simulink model "Assignment_2_3K04_Updated_2"  (R2022b)
settings: Solver=FixedStepAuto  StartTime=0.0  StopTime=1  FixedStep=1e-3  RelTol=1e-3  EnableMultiTasking=on
undefined symbols (not defined in the file): A0, A1, D0, D1, D10, D11, D12, D13, D2, D3, D4, D5, D6, D7, D8, D9, PTA0, PTA1, PTA2, PTB2, PTB23, PTB3, PTB9, PTC16, PTC17, PTC2, PTC3, PTC4, PTD0, PTD1, PTD2, PTD3
libraries: frdmk64flib x22, dspstat3 x1
settings Model: ExtModeTrigDuration=5  Creator=Stephen Oh  LastModifiedBy=Mehak
settings SolverCC: AlgebraicLoopSolver=TrustRegion
settings OptimizationCC: EnhancedBackFolding=on  PassReuseOutputArgsAs=Individual arguments  ZeroExternalMemoryAtStartup=off  ZeroInternalMemoryAtStartup=off  MaxStackSize=64  OptimizeBlockOrder=speed  DifferentSizesBufferReuse=on  OptimizationCustomize=off  EfficientTunableParamExpr=on
settings DebuggingCC: ParameterPrecisionLossMsg=none  ParameterTunabilityLossMsg=error  UnconnectedInputMsg=warning  UnconnectedOutputMsg=warning  UnconnectedLineMsg=warning  SFMachineParentedDataDiag=warning
settings HardwareCC: ProdBitPerPointer=32  ProdBitPerSizeT=32  ProdBitPerPtrDiffT=32  ProdLargestAtomicInteger=Long  ProdLargestAtomicFloat=Double  ProdWordSize=32  ProdHWDeviceType=ARM Compatible->ARM Cortex
settings ModelReferenceCC: EnableRefExpFcnMdlSchedulingChecks=on
settings SFSimCC: MATLABDynamicMemAlloc=off
settings RTWCC: Description=Embedded Coder  SystemTargetFile=ert.tlc  HardwareBoard=NXP FRDM-K64F  TLCOptions="-aInlineSetEventsForThisBaseRateFcn=TLC_FALSE -aSuppressMultiTaskScheduler=TLC_FALSE  -aRateBasedStepFcn=0"  TemplateMakefile=ert_default_tmf  Toolchain=GNU Tools for ARM Embedded Processors
settings CodeAppCC: ForceParamTrailComments=on  IgnoreCustomStorageClasses=off  OperatorAnnotations=on  SimulinkDataObjDesc=on  SFDataObjDesc=on  InsertBlockDesc=on

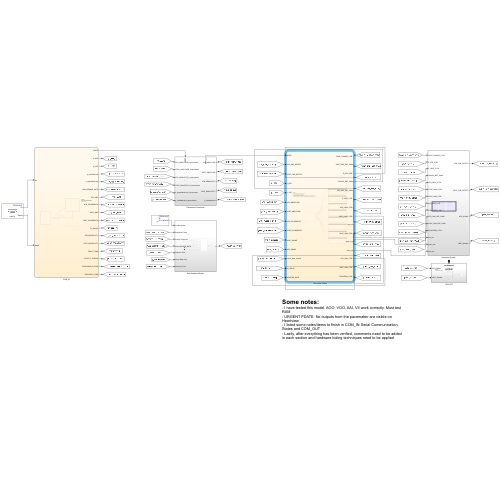
[thumbnail: Simulink's stored preview of the top-level diagram]
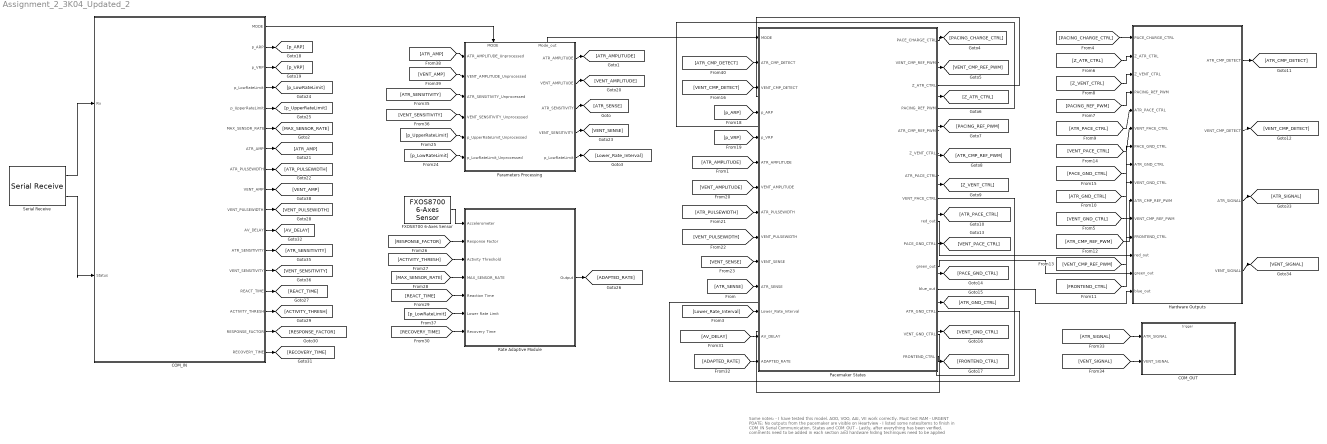
== system Assignment_2_3K04_Updated_2 ==
  note: Some notes:
      | - I have tested this model. AOO, VOO, AAI, VII work correctly. Must test RAM
      | - URGENT PDATE: No outputs from the pacemaker are visible on Heartview
      | - I listed some notes/items to finish in COM_IN Serial Communication, States and COM_OUT
      | - Lastly, after everything has been verified, comments need to be added in each section and hardware hiding techniques need to be applied
  COM_IN : Stateflow chart  TreatAsAtomicUnit=on
      settings: PortSchema="{\"entries\":[{\"content\":{\"sides\":[{\"content\":{\"connectorIds\":[\"In1\",\"In2\"]},\"type\":\"ConnectorPlacement.EquallySpacedRectSide\",\"uuid\":\"1aa50ecf-3a03-4bd0-8c8d-e8c42c1df160\"},{\"content\":{\"connectorIds\":[\"Out1\",\"Out2\",\"Out5\",\"Out3\",\"Out4\",\"Out10\",\"Out6\",\"Out9\",\"Out7\",\"Out8\",\"Out11\",\"Out17\",\"Out12\",\"Out13\",\"Out14\",\"Out15\",\"Out16\"],\"side\":\"RIGHT\"},\"type\":\"ConnectorPlacement.EquallySpacedRectSide\",\"uuid\":\"11f4d1ba-79ca-4268-a70d-42de969d73ee\"},{\"content\":{\"connectorIds\":[],\"side\":\"TOP\"},\"type\":\"ConnectorPlacement.EquallySpacedRectSide\",\"uuid\":\"6aafc352-a891-4eaa-b435-c000b57676be\"}]},\"type\":\"ConnectorPlacement.EquallySpacedConnector\",\"uuid\":\"60cf4415-29e1-4f60-bb1b-ba03cc79869a\"}],\"packageUris\":[\"http://schema.mathworks.com/mf0/Connector/R2020b\"],\"version\":\"1.0\"}"
  COM_OUT : Subsystem  TreatAsAtomicUnit=on
  FXOS8700 6-Axes Sensor : frdmk64flib/FXOS8700 6-Axes Sensor  Activesensor=Accelerometer only  ODR=800Hz  HybridODR=400Hz  Accelfullrange=-4g to +4g  SampleTime=-1
  Hardware Outputs : Subsystem
  Pacemaker States : Stateflow chart  TreatAsAtomicUnit=on
      settings: PortSchema="{\"entries\":[{\"content\":{\"sides\":[{\"content\":{\"connectorIds\":[\"In2\",\"In3\",\"In4\",\"In5\",\"In6\",\"In7\",\"In8\",\"In9\",\"In10\",\"In11\",\"In12\",\"In1\",\"In13\",\"In14\"]},\"type\":\"ConnectorPlacement.EquallySpacedRectSide\",\"uuid\":\"15e03f69-5c25-4f3e-b3fb-d71978e552f4\"},{\"content\":{\"connectorIds\":[\"Out7\",\"Out12\",\"Out4\",\"Out8\",\"Out10\",\"Out5\",\"Out9\",\"Out3\",\"Out15\",\"Out6\",\"Out14\",\"Out13\",\"Out1\",\"Out2\",\"Out11\"],\"side\":\"RIGHT\"},\"type\":\"ConnectorPlacement.EquallySpacedRectSide\",\"uuid\":\"02171bf1-edb1-4b01-9e56-a8642c556ed6\"},{\"content\":{\"connectorIds\":[],\"side\":\"TOP\"},\"type\":\"ConnectorPlacement.EquallySpacedRectSide\",\"uuid\":\"cc6b5506-3435-4740-9e3f-4dfe15d30bff\"}]},\"type\":\"ConnectorPlacement.EquallySpacedConnector\",\"uuid\":\"0ad55da7-1e65-48d0-a0a4-2620ffa94320\"}],\"packageUris\":[\"http://schema.mathworks.com/mf0/Connector/R2020b\"],\"version\":\"1.0\"}"
  Parameters Processing : Subsystem
      settings: PortSchema="{\"entries\":[{\"content\":{\"sides\":[{\"content\":{\"connectorIds\":[\"In1\",\"In2\",\"In3\",\"In4\",\"In5\",\"In6\"]},\"type\":\"ConnectorPlacement.EquallySpacedRectSide\",\"uuid\":\"651e63ca-28f2-42bd-8706-028901d11c05\"},{\"content\":{\"connectorIds\":[\"Out1\",\"Out2\",\"Out3\",\"Out4\",\"Out5\"],\"side\":\"RIGHT\"},\"type\":\"ConnectorPlacement.EquallySpacedRectSide\",\"uuid\":\"490f658c-59fe-438c-accc-92ccac1dea65\"},{\"content\":{\"connectorIds\":[\"In7\",\"Out6\"],\"side\":\"TOP\"},\"type\":\"ConnectorPlacement.EquallySpacedRectSide\",\"uuid\":\"f083c363-f6a9-47da-81a0-6b2bc7e9f843\"}]},\"type\":\"ConnectorPlacement.EquallySpacedConnector\",\"uuid\":\"6dd41c46-d50c-4376-aa14-7404fb0d5350\"}],\"packageUris\":[\"http://schema.mathworks.com/mf0/Connector/R2020b\"],\"version\":\"1.0\"}"
  Rate Adaptive Module : Subsystem
  Serial Receive : frdmk64flib/Serial Receive  SCIModule=0  Baudrate=uint32(9600)  Parity=None  StopBits=1  HardwareFlowControl=None  ByteOrder=LittleEndian  DataType=uint8  DataLength=66  BlockingMode=off  OutputStatus=on  SampleTime=-1
  wires:
  [Lower_Rate_Interval] -> Pacemaker States/1(Lower_Rate_Interval)
  [ATR_GND_CTRL] -> Hardware Outputs/8(ATR_GND_CTRL)
  [PACING_REF_PWM] -> Hardware Outputs/4(PACING_REF_PWM)
  [Z_VENT_CTRL] -> Hardware Outputs/3(Z_VENT_CTRL)
  [ATR_PACE_CTRL] -> Hardware Outputs/5(ATR_PACE_CTRL)
  Hardware Outputs/2(VENT_CMP_DETECT) -> [VENT_CMP_DETECT]
  [PACE_GND_CTRL] -> Hardware Outputs/7(PACE_GND_CTRL)
  [FRONTEND_CTRL] -> Hardware Outputs/12(FRONTEND_CTRL)
  [VENT_GND_CTRL] -> Hardware Outputs/9(VENT_GND_CTRL)
  [Z_ATR_CTRL] -> Hardware Outputs/2(Z_ATR_CTRL)
  [VENT_PACE_CTRL] -> Hardware Outputs/6(VENT_PACE_CTRL)
  [ATR_CMP_REF_PWM] -> Hardware Outputs/10(ATR_CMP_REF_PWM)
  [VENT_CMP_REF_PWM] -> Hardware Outputs/11(VENT_CMP_REF_PWM)
  [PACING_CHARGE_CTRL] -> Hardware Outputs/1(PACE_CHARGE_CTRL)
  Hardware Outputs/1(ATR_CMP_DETECT) -> [ATR_CMP_DETECT]
  [VENT_CMP_DETECT] -> Pacemaker States/4(VENT_CMP_DETECT)
  [p_ARP] -> Pacemaker States/5(p_ARP)
  [p_VRP] -> Pacemaker States/6(p_VRP)
  [ATR_CMP_DETECT] -> Pacemaker States/3(ATR_CMP_DETECT)
  [ATR_AMPLITUDE] -> Pacemaker States/7(ATR_AMPLITUDE)
  [VENT_AMPLITUDE] -> Pacemaker States/8(VENT_AMPLITUDE)
  [ATR_PULSEWIDTH] -> Pacemaker States/9(ATR_PULSEWIDTH)
  [VENT_PULSEWIDTH] -> Pacemaker States/10(VENT_PULSEWIDTH)
  Parameters Processing/1(ATR_AMPLITUDE) -> [ATR_AMPLITUDE]
  Parameters Processing/5(p_LowRateLimit) -> [Lower_Rate_Interval]
  Pacemaker States/3(VENT_PACE_CTRL) -> [VENT_PACE_CTRL]
  Pacemaker States/9(ATR_PACE_CTRL) -> [ATR_PACE_CTRL]
  Pacemaker States/7(PACE_CHARGE_CTRL) -> [PACING_CHARGE_CTRL]
  Pacemaker States/12(VENT_CMP_REF_PWM) -> [VENT_CMP_REF_PWM]
  Pacemaker States/4(Z_ATR_CTRL) -> [Z_ATR_CTRL]
  Pacemaker States/8(PACING_REF_PWM) -> [PACING_REF_PWM]
  Pacemaker States/10(ATR_CMP_REF_PWM) -> [ATR_CMP_REF_PWM]
  Pacemaker States/5(Z_VENT_CTRL) -> [Z_VENT_CTRL]
  Pacemaker States/6(PACE_GND_CTRL) -> [PACE_GND_CTRL]
  Pacemaker States/1(ATR_GND_CTRL) -> [ATR_GND_CTRL]
  Pacemaker States/2(VENT_GND_CTRL) -> [VENT_GND_CTRL]
  Pacemaker States/11(FRONTEND_CTRL) -> [FRONTEND_CTRL]
  [ATR_SENSE] -> Pacemaker States/12(ATR_SENSE)
  [VENT_SENSE] -> Pacemaker States/11(VENT_SENSE)
  Serial Receive/1 -> COM_IN/1(Rx)
  Serial Receive/2 -> COM_IN/2(Status)
  COM_IN/1(MODE) -> Parameters Processing/7(MODE)
  Parameters Processing/6(Mode_out) -> Pacemaker States/2(MODE)
  Parameters Processing/2(VENT_AMPLITUDE) -> [VENT_AMPLITUDE]
  [p_UpperRateLimit] -> Parameters Processing/5(p_UpperRateLimit_Unprocessed)
  COM_IN/11(AV_DELAY) -> [AV_DELAY]
  [AV_DELAY] -> Pacemaker States/13(AV_DELAY)
  [ADAPTED_RATE] -> Pacemaker States/14(ADAPTED_RATE)
  Parameters Processing/3(ATR_SENSITIVITY) -> [ATR_SENSE]
  Parameters Processing/4(VENT_SENSITIVITY) -> [VENT_SENSE]
  FXOS8700 6-Axes Sensor/1 -> Rate Adaptive Module/1(Accelerometer)
  Rate Adaptive Module/1(Output) -> [ADAPTED_RATE]
  [RESPONSE_FACTOR] -> Rate Adaptive Module/2(Response Factor)
  [ACTIVITY_THRESH] -> Rate Adaptive Module/3(Activity Threshold)
  [MAX_SENSOR_RATE] -> Rate Adaptive Module/4(MAX_SENSOR_RATE)
  [REACT_TIME] -> Rate Adaptive Module/5(Reaction Time)
  [p_LowRateLimit] -> Parameters Processing/6(p_LowRateLimit_Unprocessed)
  [RECOVERY_TIME] -> Rate Adaptive Module/7(Recovery Time)
  Hardware Outputs/3(ATR_SIGNAL) -> [ATR_SIGNAL]
  Hardware Outputs/4(VENT_SIGNAL) -> [VENT_SIGNAL]
  [ATR_SIGNAL] -> COM_OUT/1(ATR_SIGNAL)
  [VENT_SIGNAL] -> COM_OUT/2(VENT_SIGNAL)
  [ATR_SENSITIVITY] -> Parameters Processing/3(ATR_SENSITIVITY_Unprocessed)
  [VENT_SENSITIVITY] -> Parameters Processing/4(VENT_SENSITIVITY_Unprocessed)
  [p_LowRateLimit] -> Rate Adaptive Module/6(Lower Rate Limit)
  COM_IN/3(p_LowRateLimit) -> [p_LowRateLimit]
  COM_IN/4(p_UpperRateLimit) -> [p_UpperRateLimit]
  COM_IN/5(p_VRP) -> [p_VRP]
  COM_IN/2(p_ARP) -> [p_ARP]
  COM_IN/10(MAX_SENSOR_RATE) -> [MAX_SENSOR_RATE]
  COM_IN/17(ATR_SENSITIVITY) -> [ATR_SENSITIVITY]
  COM_IN/12(VENT_SENSITIVITY) -> [VENT_SENSITIVITY]
  COM_IN/9(ATR_PULSEWIDTH) -> [ATR_PULSEWIDTH]
  COM_IN/8(VENT_PULSEWIDTH) -> [VENT_PULSEWIDTH]
  COM_IN/6(ATR_AMP) -> [ATR_AMP]
  COM_IN/7(VENT_AMP) -> [VENT_AMP]
  COM_IN/13(REACT_TIME) -> [REACT_TIME]
  COM_IN/14(ACTIVITY_THRESH) -> [ACTIVITY_THRESH]
  COM_IN/15(RESPONSE_FACTOR) -> [RESPONSE_FACTOR]
  COM_IN/16(RECOVERY_TIME) -> [RECOVERY_TIME]
  [ATR_AMP] -> Parameters Processing/1(ATR_AMPLITUDE_Unprocessed)
  [VENT_AMP] -> Parameters Processing/2(VENT_AMPLITUDE_Unprocessed)
  Pacemaker States/15(red_out) -> Hardware Outputs/13(red_out)
  Pacemaker States/13(blue_out) -> Hardware Outputs/15(blue_out)
  Pacemaker States/14(green_out) -> Hardware Outputs/14(green_out)

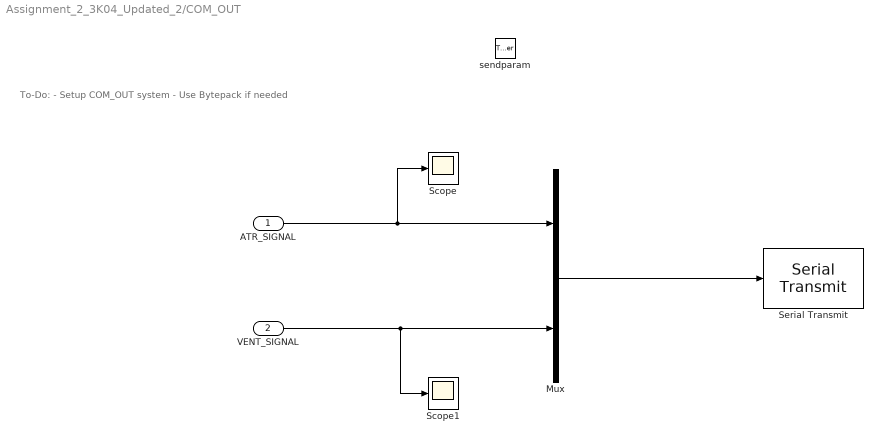
== system Assignment_2_3K04_Updated_2/COM_OUT ==
  note: To-Do:
      | - Setup COM_OUT system
      | - Use Bytepack if needed
  ATR_SIGNAL : Inport  OutDataTypeStr=double
  VENT_SIGNAL : Inport  Port=2  OutDataTypeStr=double
  sendparam : TriggerPort  TriggerType=function-call  IsSimulinkFunction=on  FunctionName=sendparam  VariantControl=(inherit)  PortDimensions=1
  Mux : Mux  Inputs=2
  Scope : Scope
  Scope1 : Scope
  Serial Transmit : frdmk64flib/Serial Transmit  SCIModule=0  Baudrate=uint32(9600)  Parity=None  StopBits=1  HardwareFlowControl=None  ByteOrder=LittleEndian  BlockingMode=on  OutputStatus=off
  wires:
  ATR_SIGNAL/1 -> Scope/1, Mux/1
  VENT_SIGNAL/1 -> Scope1/1, Mux/2
  Mux/1 -> Serial Transmit/1

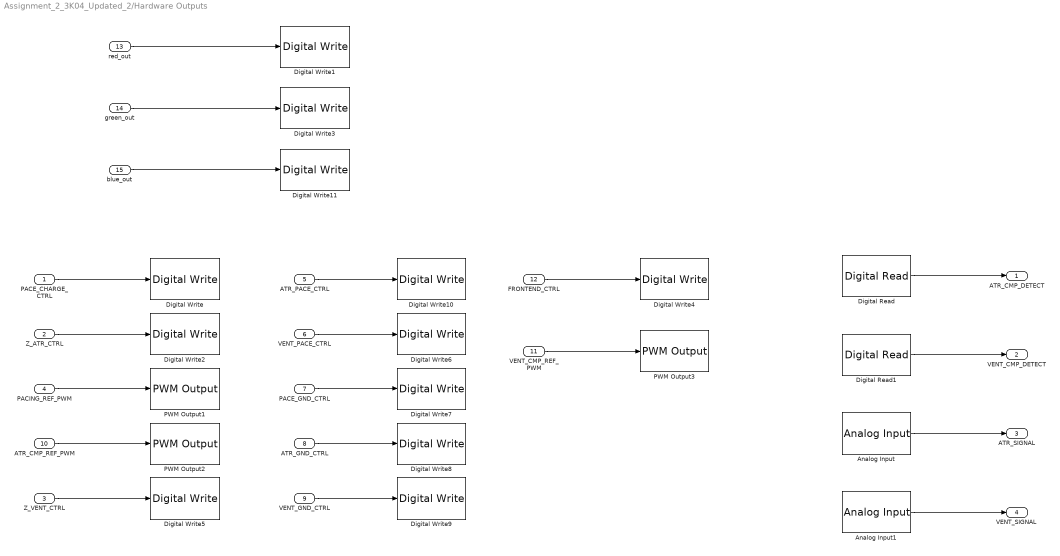
== system Assignment_2_3K04_Updated_2/Hardware Outputs ==
  PACE_CHARGE_CTRL : Inport
  Z_ATR_CTRL : Inport  Port=2
  Z_VENT_CTRL : Inport  Port=3
  PACING_REF_PWM : Inport  Port=4
  ATR_PACE_CTRL : Inport  Port=5
  VENT_PACE_CTRL : Inport  Port=6
  PACE_GND_CTRL : Inport  Port=7
  ATR_GND_CTRL : Inport  Port=8
  VENT_GND_CTRL : Inport  Port=9
  ATR_CMP_REF_PWM : Inport  Port=10
  VENT_CMP_REF_PWM : Inport  Port=11
  FRONTEND_CTRL : Inport  Port=12
  red_out : Inport  Port=13
  green_out : Inport  Port=14
  blue_out : Inport  Port=15
  Analog Input : frdmk64flib/Analog Input  Whichpin=PTB2 (A0)  SampleTime=-1
  Analog Input1 : frdmk64flib/Analog Input  Whichpin=PTB3 (A1)  SampleTime=-1
  Digital Read : frdmk64flib/Digital Read  Whichpin=PTC16 (D0)  SampleTime=-1
  Digital Read1 : frdmk64flib/Digital Read  Whichpin=PTC17 (D1)  SampleTime=-1
  Digital Write : frdmk64flib/Digital Write  Whichpin=PTB9 (D2)
  Digital Write1 : frdmk64flib/Digital Write  Whichpin=RED_LED
  Digital Write10 : frdmk64flib/Digital Write  Whichpin=PTA0 (D8)
  Digital Write11 : frdmk64flib/Digital Write  Whichpin=BLUE_LED
  Digital Write2 : frdmk64flib/Digital Write  Whichpin=PTB23 (D4)
  Digital Write3 : frdmk64flib/Digital Write  Whichpin=GREEN_LED
  Digital Write4 : frdmk64flib/Digital Write  Whichpin=PTD1 (D13)
  Digital Write5 : frdmk64flib/Digital Write  Whichpin=PTC3 (D7)
  Digital Write6 : frdmk64flib/Digital Write  Whichpin=PTC4 (D9)
  Digital Write7 : frdmk64flib/Digital Write  Whichpin=PTD0 (D10)
  Digital Write8 : frdmk64flib/Digital Write  Whichpin=PTD2 (D11)
  Digital Write9 : frdmk64flib/Digital Write  Whichpin=PTD3 (D12)
  PWM Output1 : frdmk64flib/PWM Output  Whichpin=PTA2 (D5)  InitialFrequency=2000  InitialDutyCycle=0
  PWM Output2 : frdmk64flib/PWM Output  Whichpin=PTC2 (D6)  InitialFrequency=2000  InitialDutyCycle=0
  PWM Output3 : frdmk64flib/PWM Output  Whichpin=PTA1 (D3)  InitialFrequency=2000  InitialDutyCycle=0
  ATR_CMP_DETECT : Outport
  VENT_CMP_DETECT : Outport  Port=2
  ATR_SIGNAL : Outport  Port=3  OutDataTypeStr=double
  VENT_SIGNAL : Outport  Port=4  OutDataTypeStr=double
  wires:
  Analog Input1/1 -> VENT_SIGNAL/1
  Analog Input/1 -> ATR_SIGNAL/1
  FRONTEND_CTRL/1 -> Digital Write4/1
  Digital Read1/1 -> VENT_CMP_DETECT/1
  PACE_GND_CTRL/1 -> Digital Write7/1
  VENT_CMP_REF_PWM/1 -> PWM Output3/1
  Z_VENT_CTRL/1 -> Digital Write5/1
  PACE_CHARGE_CTRL/1 -> Digital Write/1
  PACING_REF_PWM/1 -> PWM Output1/1
  ATR_GND_CTRL/1 -> Digital Write8/1
  VENT_PACE_CTRL/1 -> Digital Write6/1
  ATR_CMP_REF_PWM/1 -> PWM Output2/1
  VENT_GND_CTRL/1 -> Digital Write9/1
  Digital Read/1 -> ATR_CMP_DETECT/1
  Z_ATR_CTRL/1 -> Digital Write2/1
  ATR_PACE_CTRL/1 -> Digital Write10/1
  blue_out/1 -> Digital Write11/1
  red_out/1 -> Digital Write1/1
  green_out/1 -> Digital Write3/1

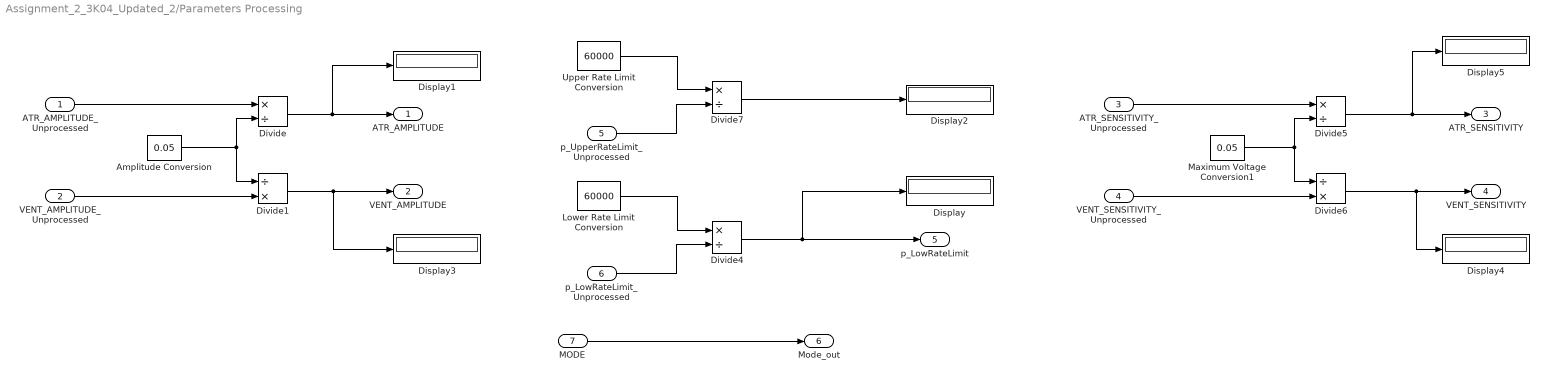
== system Assignment_2_3K04_Updated_2/Parameters Processing ==
  ATR_AMPLITUDE_Unprocessed : Inport  OutDataTypeStr=single
  VENT_AMPLITUDE_Unprocessed : Inport  Port=2  OutDataTypeStr=single
  ATR_SENSITIVITY_Unprocessed : Inport  Port=3  OutDataTypeStr=single
  VENT_SENSITIVITY_Unprocessed : Inport  Port=4  OutDataTypeStr=single
  p_UpperRateLimit_Unprocessed : Inport  Port=5  OutDataTypeStr=single
  p_LowRateLimit_Unprocessed : Inport  Port=6  OutDataTypeStr=single
  MODE : Inport  Port=7
  Amplitude Conversion : Constant  Value=0.05  OutDataTypeStr=single
  Display{,1..5} (6 alike) : Display
  Divide : Product  Inputs=*/  OutDataTypeStr=single
  Divide1 : Product  Inputs=/*  OutDataTypeStr=single
  Divide4 : Product  Inputs=*/  OutDataTypeStr=single  RndMeth=Nearest
  Divide5 : Product  Inputs=*/  OutDataTypeStr=single
  Divide6 : Product  Inputs=/*  OutDataTypeStr=single
  Divide7 : Product  Inputs=*/  OutDataTypeStr=single  RndMeth=Nearest
  Lower Rate Limit Conversion : Constant  Value=60000  OutDataTypeStr=single
  Maximum Voltage Conversion1 : Constant  Value=0.05  OutDataTypeStr=single
  Upper Rate Limit Conversion : Constant  Value=60000  OutDataTypeStr=single
  ATR_AMPLITUDE : Outport  OutDataTypeStr=single
  VENT_AMPLITUDE : Outport  Port=2  OutDataTypeStr=single
  ATR_SENSITIVITY : Outport  Port=3  OutDataTypeStr=single
  VENT_SENSITIVITY : Outport  Port=4  OutDataTypeStr=single
  p_LowRateLimit : Outport  Port=5  OutDataTypeStr=single
  Mode_out : Outport  Port=6
  wires:
  Divide5/1 -> Display5/1, ATR_SENSITIVITY/1
  Divide7/1 -> Display2/1
  Upper Rate Limit Conversion/1 -> Divide7/1
  p_UpperRateLimit_Unprocessed/1 -> Divide7/2
  Lower Rate Limit Conversion/1 -> Divide4/1
  Divide1/1 -> Display3/1, VENT_AMPLITUDE/1
  ATR_SENSITIVITY_Unprocessed/1 -> Divide5/1
  p_LowRateLimit_Unprocessed/1 -> Divide4/2
  Maximum Voltage Conversion1/1 -> Divide6/1, Divide5/2
  Divide/1 -> Display1/1, ATR_AMPLITUDE/1
  Divide4/1 -> p_LowRateLimit/1, Display/1
  VENT_AMPLITUDE_Unprocessed/1 -> Divide1/2
  VENT_SENSITIVITY_Unprocessed/1 -> Divide6/2
  ATR_AMPLITUDE_Unprocessed/1 -> Divide/1
  Divide6/1 -> Display4/1, VENT_SENSITIVITY/1
  Amplitude Conversion/1 -> Divide1/1, Divide/2
  MODE/1 -> Mode_out/1

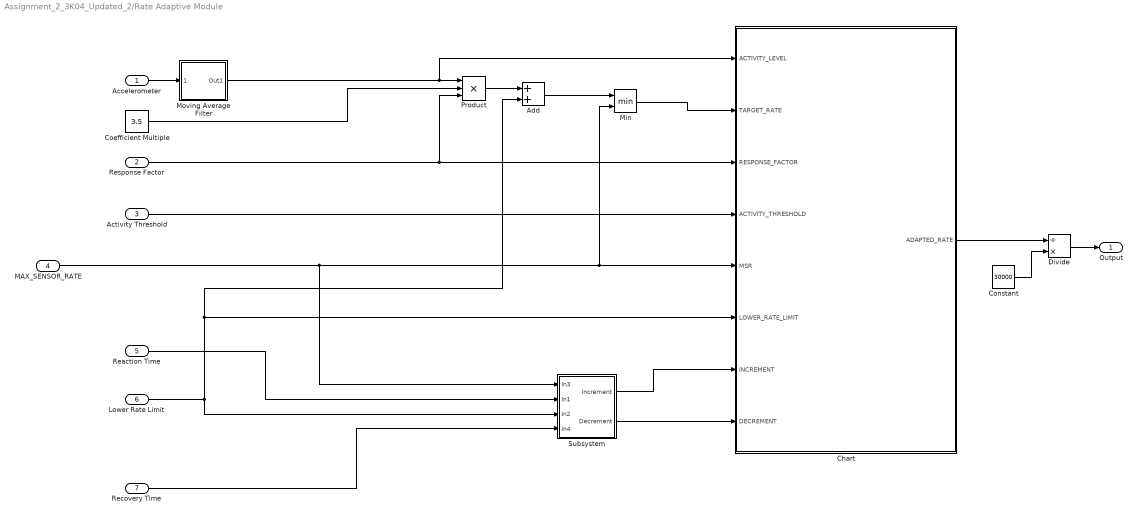
== system Assignment_2_3K04_Updated_2/Rate Adaptive Module ==
  Accelerometer : Inport
  Response Factor : Inport  Port=2
  Activity Threshold : Inport  Port=3
  MAX_SENSOR_RATE : Inport  Port=4
  Reaction Time : Inport  Port=5
  Lower Rate Limit : Inport  Port=6
  Recovery Time : Inport  Port=7
  Add : Sum
  Chart : Stateflow chart  TreatAsAtomicUnit=on
      settings: PortSchema="{\"entries\":[{\"content\":{\"sides\":[{\"content\":{\"connectorIds\":[\"In1\",\"In3\",\"In2\",\"In6\",\"In8\",\"In7\",\"In4\",\"In5\"]},\"type\":\"ConnectorPlacement.EquallySpacedRectSide\",\"uuid\":\"efebee7e-2c09-4b25-ba04-904f72c011ed\"},{\"content\":{\"connectorIds\":[\"Out1\"],\"side\":\"RIGHT\"},\"type\":\"ConnectorPlacement.EquallySpacedRectSide\",\"uuid\":\"6322cc63-1b7a-423a-b49b-7b27e71e0c32\"},{\"content\":{\"connectorIds\":[],\"side\":\"TOP\"},\"type\":\"ConnectorPlacement.EquallySpacedRectSide\",\"uuid\":\"daf2dbd4-7676-46e9-bb01-958bd0e2e14e\"}]},\"type\":\"ConnectorPlacement.EquallySpacedConnector\",\"uuid\":\"43c3c7b3-b94c-45f5-b310-1a430cfb2b71\"}],\"packageUris\":[\"http://schema.mathworks.com/mf0/Connector/19700101\"],\"version\":\"1.0\"}"
  Coefficient Multiple : Constant  Value=3.5
  Constant : Constant  Value=30000
  Divide : Product  Inputs=/*
  Min : MinMax  Inputs=2
  Moving Average Filter : Subsystem
  Product : Product  Inputs=3
  Subsystem : Subsystem
  Output : Outport
  wires:
  Recovery Time/1 -> Subsystem/4(In4)
  MAX_SENSOR_RATE/1 -> Subsystem/1(In3), Min/2, Chart/8(MSR)
  Subsystem/1(Increment) -> Chart/4(INCREMENT)
  Activity Threshold/1 -> Chart/6(ACTIVITY_THRESHOLD)
  Response Factor/1 -> Product/3, Chart/2(RESPONSE_FACTOR)
  Lower Rate Limit/1 -> Subsystem/3(In2), Chart/7(LOWER_RATE_LIMIT), Add/2
  Add/1 -> Min/1
  Product/1 -> Add/1
  Min/1 -> Chart/3(TARGET_RATE)
  Reaction Time/1 -> Subsystem/2(In1)
  Subsystem/2(Decrement) -> Chart/5(DECREMENT)
  Chart/1(ADAPTED_RATE) -> Divide/1
  Coefficient Multiple/1 -> Product/2
  Divide/1 -> Output/1
  Constant/1 -> Divide/2
  Moving Average Filter/1(Out1) -> Chart/1(ACTIVITY_LEVEL), Product/1
  Accelerometer/1 -> Moving Average Filter/1(Accelerometer)

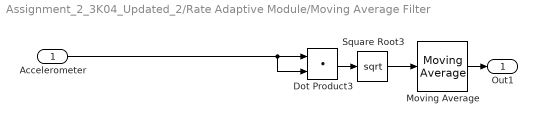
== system Assignment_2_3K04_Updated_2/Rate Adaptive Module/Moving Average Filter ==
  Accelerometer : Inport
  Dot Product3 : DotProduct  OutDataTypeStr=Inherit: Inherit via internal rule
  Moving Average : dspstat3/Moving Average  Method=Sliding window  ForgettingFactorPort=off  SpecifyWindowLength=on  WindowLength=500  OverlapLength=499  AllowArbitraryInputLength=off  ForgettingFactor=0.9  SimulateUsing=Code generation
  Square Root3 : Sqrt
  Out1 : Outport
  wires:
  Accelerometer/1 -> Dot Product3/2, Dot Product3/1
  Dot Product3/1 -> Square Root3/1
  Square Root3/1 -> Moving Average/1
  Moving Average/1 -> Out1/1

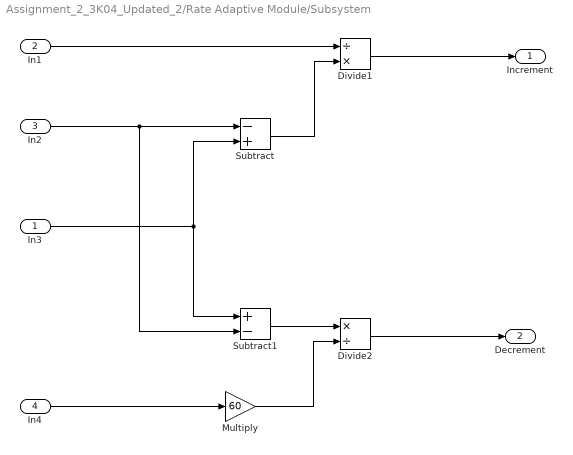
== system Assignment_2_3K04_Updated_2/Rate Adaptive Module/Subsystem ==
  In3 : Inport  OutDataTypeStr=single
  In1 : Inport  Port=2  OutDataTypeStr=single
  In2 : Inport  Port=3  OutDataTypeStr=single
  In4 : Inport  Port=4  OutDataTypeStr=single
  Divide1 : Product  Inputs=/*  RndMeth=Ceiling
  Divide2 : Product  Inputs=*/  RndMeth=Ceiling  SaturateOnIntegerOverflow=on
  Multiply : Gain  Gain=60
  Subtract : Sum  Inputs=-+
  Subtract1 : Sum  Inputs=+-
  Increment : Outport  OutDataTypeStr=single
  Decrement : Outport  Port=2  OutDataTypeStr=single
  wires:
  Multiply/1 -> Divide2/2
  In2/1 -> Subtract1/2, Subtract/1
  In3/1 -> Subtract/2, Subtract1/1
  Divide1/1 -> Increment/1
  In1/1 -> Divide1/1
  Subtract1/1 -> Divide2/1
  Subtract/1 -> Divide1/2
  In4/1 -> Multiply/1
  Divide2/1 -> Decrement/1

== stateflow chart Assignment_2_3K04_Updated_2/COM_IN ==
  state SET_PARAM
    % Uses serial input to assign values to the parameters
    entry:
    MODE = Rx(1);
    p_ARP = typecast(Rx(2:5), "single");
    p_VRP = typecast(Rx(6:9), "single");
    p_LowRateLimit = typecast(Rx(10:13), "single");
    p_UpperRateLimit = typecast(Rx(14:17), "single");
    MAX_SENSOR_RATE = typecast(Rx(18:21), "single");
    ATR_AMP = typecast(Rx(22:25), "single");
    ATR_PULSEWIDTH = typecast(Rx(26:29), "single");
    VENT_AMP = typecast(Rx(30:33), "single");
    VENT_PULSEWIDTH = typecast(Rx(34:37), "single");
    AV_DELAY = typecast(Rx(38:41), "single");
    ATR_SENSITIVITY = typecast(Rx(42:45), "single");
    VENT_SENSITIVITY = typecast(Rx(46:49), "single");
    REACT_TIME = typecast(Rx(50:53), "single");
    ACTIVITY_THRESH = typecast(Rx(54:57), "single");
    RESPONSE_FACTOR = typecast(Rx(58:61), "single");
    RECOVERY_TIME = typecast(Rx(62:65), "single");
  note: To-Do:
      | - Set number of transmitted bytes
      | - Update SET_PARAM with values
      | - Verify Fuction
  state INITIAL
    % Set the initial values of parameters
    entry:
    MODE = 5;
    p_ARP = 250;
    p_VRP = 320;
    p_LowRateLimit = 60;
    p_UpperRateLimit = 120;
    MAX_SENSOR_RATE = 120;
    ATR_AMP = 3.5;
    ATR_PULSEWIDTH = 1;
    VENT_AMP = 3.5;
    VENT_PULSEWIDTH = 1;
    AV_DELAY = 150;
    ATR_SENSITIVITY = 4;
    VENT_SENSITIVITY = 4;
    REACT_TIME = 30;
    ACTIVITY_THRESH = 1.1;
    RESPONSE_FACTOR = 8;
    RECOVERY_TIME = 5;
  state STANDBY
    % Wait for COM
  state ECHO_PARAM [commented out]
    entry:
    % Sends back the current value of the parameters
    sendparam();
  SET_PARAM -> STANDBY
  (default) -> INITIAL
  (junction 13) -> SET_PARAM : [Rx(66) == hex2dec('00')]
  (junction 12) -> STANDBY [order 2]
  INITIAL -> STANDBY
  STANDBY -> (junction 12) : [Status == 0]
  (junction 12) -> (junction 13) [order 1]
  (junction 13) -> ECHO_PARAM [commented out] : [Rx(2) == hex2dec('22')]
  ECHO_PARAM -> STANDBY [commented out]
  data: Rx input uint8; Status input uint8; MODE output uint8; p_ARP output single; p_LowRateLimit output single; p_UpperRateLimit output single; p_VRP output single; ATR_AMP output single; VENT_AMP output single; VENT_PULSEWIDTH output single; ATR_PULSEWIDTH output single; MAX_SENSOR_RATE output single; AV_DELAY output single; VENT_SENSITIVITY output single; REACT_TIME output single; ACTIVITY_THRESH output single; RESPONSE_FACTOR output single; RECOVERY_TIME output single; ATR_SENSITIVITY output single

== stateflow chart Assignment_2_3K04_Updated_2/Rate Adaptive Module/Chart ==
  state RateSelect
    entry:
    ADAPTED_RATE = LOWER_RATE_LIMIT
  state Increment
    entry:
    ADAPTED_RATE = ADAPTED_RATE + INCREMENT
  state TargetRateAchieved
  state Decrement
    entry:
    ADAPTED_RATE = ADAPTED_RATE - DECREMENT
  Increment -> Increment [order 2] : after(1000, msec) [ACTIVITY_LEVEL > ACTIVITY_THRESHOLD]
  (default) -> RateSelect
  Increment -> TargetRateAchieved [order 1] : [ADAPTED_RATE >= TARGET_RATE ]
  RateSelect -> Increment [order 1] : [ACTIVITY_LEVEL > ACTIVITY_THRESHOLD]
  RateSelect -> RateSelect [order 2] : [ACTIVITY_LEVEL < ACTIVITY_THRESHOLD]
  Decrement -> RateSelect [order 3] : [ADAPTED_RATE <= LOWER_RATE_LIMIT]
  Decrement -> Increment [order 1] : after(1000, msec) [ACTIVITY_LEVEL > ACTIVITY_THRESHOLD]
  Increment -> Decrement [order 3] : after(1000, msec) [ACTIVITY_LEVEL < ACTIVITY_THRESHOLD]
  TargetRateAchieved -> Decrement : [ACTIVITY_LEVEL < ACTIVITY_THRESHOLD]
  Decrement -> Decrement [order 2] : after(1000, msec) [ACTIVITY_LEVEL < ACTIVITY_THRESHOLD]
  data: ACTIVITY_LEVEL input; RESPONSE_FACTOR input; ADAPTED_RATE output; TARGET_RATE input; INCREMENT input; DECREMENT input; ACTIVITY_THRESHOLD input; LOWER_RATE_LIMIT input; MSR input

== stateflow chart Assignment_2_3K04_Updated_2/Pacemaker States ==
  state AOO
    state Charging
      entry:
      %
      % Charging capacitor C22
      ATR_PACE_CTRL = LOW
      VENT_PACE_CTRL = LOW
      PACING_REF_PWM = ATR_AMPLITUDE
      PACE_CHARGE_CTRL = HIGH
      %
      % Release of capacitor C21 into ground
      PACE_GND_CTRL = HIGH
      VENT_PACE_CTRL = LOW
      Z_ATR_CTRL = LOW
      Z_VENT_CTRL = LOW
      ATR_PACE_CTRL = LOW
      ATR_GND_CTRL = HIGH
      VENT_GND_CTRL = LOW
      red_out = 1;
      green_out = 0;
      blue_out = 0;
    state Discharging
      entry:
      %
      % Charge release of capacitor C22 into C21
      PACE_CHARGE_CTRL = LOW
      PACE_GND_CTRL = HIGH
      VENT_PACE_CTRL = LOW
      VENT_GND_CTRL = LOW
      Z_VENT_CTRL = LOW
      Z_ATR_CTRL = LOW
      ATR_GND_CTRL = LOW
      ATR_PACE_CTRL = HIGH
    (default) -> AOO.Charging
    AOO.Charging -> AOO.Discharging : after(delayINTERVAL, msec)
    AOO.Discharging -> AOO.Charging : after(delayATR_PULSEWIDTH, msec)
  note: To-Do:
      | - AOO, VOO, AAI, VVI work as intended
      | - Uncertain about AOOR and VOOR
      | - AAIR and VVIR work as intended (double-check on another pacemaker)
      | - Finally, add comments + organize
      | - If there is enough time remaining, implement DDDR (else delete AV_DELAY)
  state VOO
    state Charging
      entry:
      %
      % Charging capacitor C22
      ATR_PACE_CTRL = LOW
      VENT_PACE_CTRL = LOW
      PACING_REF_PWM = VENT_AMPLITUDE
      PACE_CHARGE_CTRL = HIGH
      %
      % Charge release of capacitor C21 into ground
      PACE_GND_CTRL = HIGH
      VENT_PACE_CTRL = LOW
      Z_ATR_CTRL = LOW
      Z_VENT_CTRL = LOW
      ATR_PACE_CTRL = LOW
      ATR_GND_CTRL = LOW
      VENT_GND_CTRL = HIGH
      red_out = 0;
      green_out = 0;
      blue_out = 1;
    state Discharging
      entry:
      %
      % Charge release of capacitor C22 into C21
      PACE_CHARGE_CTRL = LOW
      PACE_GND_CTRL = HIGH
      ATR_PACE_CTRL = LOW
      ATR_GND_CTRL = LOW
      Z_VENT_CTRL = LOW
      Z_ATR_CTRL = LOW
      VENT_GND_CTRL = LOW
      VENT_PACE_CTRL = HIGH
    (default) -> VOO.Charging
    VOO.Charging -> VOO.Discharging : after(delayINTERVAL, msec)
    VOO.Discharging -> VOO.Charging : after(delayVENT_PULSEWIDTH, msec)
  state AAI
    state Transition
      % Check for intrinsic pulse
    state Discharging
      entry:
      %
      % Charge release of capacitor C22 into C21
      PACE_CHARGE_CTRL = LOW
      PACE_GND_CTRL = HIGH
      VENT_PACE_CTRL = LOW
      VENT_GND_CTRL = LOW
      Z_VENT_CTRL = LOW
      Z_ATR_CTRL = LOW
      ATR_GND_CTRL = LOW
      ATR_PACE_CTRL = HIGH
    state Charging
      entry:
      %
      % Turn sensing on
      FRONTEND_CTRL = HIGH
      ATR_CMP_REF_PWM = ATR_SENSE
      %
      % Charging capacitor C22
      ATR_PACE_CTRL = LOW
      VENT_PACE_CTRL = LOW
      PACING_REF_PWM = ATR_AMPLITUDE
      PACE_CHARGE_CTRL = HIGH
      %
      % Charge release of capacitor C21 into ground
      PACE_GND_CTRL = HIGH
      VENT_PACE_CTRL = LOW
      Z_ATR_CTRL = LOW
      Z_VENT_CTRL = LOW
      ATR_PACE_CTRL = LOW
      ATR_GND_CTRL = HIGH
      VENT_GND_CTRL = LOW
    AAI.Transition -> AAI.Discharging [order 1] : after(delayINTERVAL-delayARP, msec)
    AAI.Transition -> AAI.Charging [order 2] : [ATR_CMP_DETECT == HIGH]
    AAI.Charging -> AAI.Transition : after(delayARP, msec)
    (default) -> AAI.Charging
    AAI.Discharging -> AAI.Charging : after(delayATR_PULSEWIDTH, msec)
  state VVI
    state Transition
      % Check for intrinsic pulse
    state Charging
      entry:
      %
      % Turn sensing on
      FRONTEND_CTRL = HIGH
      VENT_CMP_REF_PWM = VENT_SENSE
      %
      % Charging capacitor C22
      ATR_PACE_CTRL = LOW
      VENT_PACE_CTRL = LOW
      PACING_REF_PWM = VENT_AMPLITUDE
      PACE_CHARGE_CTRL = HIGH
      %
      % Charge release of capacitor C21 into ground
      PACE_GND_CTRL = HIGH
      VENT_PACE_CTRL = LOW
      Z_ATR_CTRL = LOW
      Z_VENT_CTRL = LOW
      ATR_PACE_CTRL = LOW
      ATR_GND_CTRL = LOW
      VENT_GND_CTRL = HIGH
    state Discharging
      entry:
      %
      % Charge release of capacitor C22 into C21
      PACE_CHARGE_CTRL = LOW
      PACE_GND_CTRL = HIGH
      ATR_PACE_CTRL = LOW
      ATR_GND_CTRL = LOW
      Z_VENT_CTRL = LOW
      Z_ATR_CTRL = LOW
      VENT_GND_CTRL = LOW
      VENT_PACE_CTRL = HIGH
    VVI.Transition -> VVI.Discharging [order 1] : after(delayINTERVAL-delayVRP, msec)
    VVI.Transition -> VVI.Charging [order 2] : [VENT_CMP_DETECT == HIGH]
    VVI.Charging -> VVI.Transition : after(delayVRP, msec)
    (default) -> VVI.Charging
    VVI.Discharging -> VVI.Charging : after(delayVENT_PULSEWIDTH, msec)
  state ModeSelect
  state AOOR
    state Charging
      entry:
      %
      % Charging capacitor C22
      ATR_PACE_CTRL = LOW
      VENT_PACE_CTRL = LOW
      PACING_REF_PWM = ATR_AMPLITUDE
      PACE_CHARGE_CTRL = HIGH
      %
      % Charge release of capacitor C21 into ground
      PACE_GND_CTRL = HIGH
      VENT_PACE_CTRL = LOW
      Z_ATR_CTRL = LOW
      Z_VENT_CTRL = LOW
      ATR_PACE_CTRL = LOW
      ATR_GND_CTRL = HIGH
      VENT_GND_CTRL = LOW
    state Discharging
      entry:
      %
      %Charge release of capacitor C22 into C21
      PACE_CHARGE_CTRL = LOW
      PACE_GND_CTRL = HIGH
      VENT_PACE_CTRL = LOW
      VENT_GND_CTRL = LOW
      Z_VENT_CTRL = LOW
      Z_ATR_CTRL = LOW
      ATR_GND_CTRL = LOW
      ATR_PACE_CTRL = HIGH
    (default) -> AOOR.Charging
    AOOR.Charging -> AOOR.Discharging : after(ADAPTED_RATE, msec)
    AOOR.Discharging -> AOOR.Charging : after(delayATR_PULSEWIDTH, msec)
  state VOOR
    state Discharging
      entry:
      %
      % Charge release of capacitor C22 into C21
      PACE_CHARGE_CTRL = LOW
      PACE_GND_CTRL = HIGH
      ATR_PACE_CTRL = LOW
      ATR_GND_CTRL = LOW
      Z_VENT_CTRL = LOW
      Z_ATR_CTRL = LOW
      VENT_GND_CTRL = LOW
      VENT_PACE_CTRL = HIGH
    state Charging
      entry:
      %
      % Charging capacitor C22
      ATR_PACE_CTRL = LOW
      VENT_PACE_CTRL = LOW
      PACING_REF_PWM = VENT_AMPLITUDE
      PACE_CHARGE_CTRL = HIGH
      %
      % Charge release of capacitor C21 into ground
      PACE_GND_CTRL = HIGH
      VENT_PACE_CTRL = LOW
      Z_ATR_CTRL = LOW
      Z_VENT_CTRL = LOW
      ATR_PACE_CTRL = LOW
      ATR_GND_CTRL = LOW
      VENT_GND_CTRL = HIGH
      red_out = 0;
      green_out = 1;
      blue_out = 0;
    (default) -> VOOR.Charging
    VOOR.Charging -> VOOR.Discharging : after(ADAPTED_RATE, msec)
    VOOR.Discharging -> VOOR.Charging : after(delayVENT_PULSEWIDTH, msec)
  state AAIR
    state Transition
      % Check for intrinsic pulse
    state Discharging
      entry:
      %
      % Charge release of capacitor C22 into C21
      PACE_CHARGE_CTRL = LOW
      PACE_GND_CTRL = HIGH
      VENT_PACE_CTRL = LOW
      VENT_GND_CTRL = LOW
      Z_VENT_CTRL = LOW
      Z_ATR_CTRL = LOW
      ATR_GND_CTRL = LOW
      ATR_PACE_CTRL = HIGH
    state Charging
      entry:
      %
      % Turn sensing on
      FRONTEND_CTRL = HIGH
      ATR_CMP_REF_PWM = ATR_SENSE
      %
      % Charging capacitor C22
      ATR_PACE_CTRL = LOW
      VENT_PACE_CTRL = LOW
      PACING_REF_PWM = ATR_AMPLITUDE
      PACE_CHARGE_CTRL = HIGH
      %
      % Charge release of capacitor C21 into ground
      PACE_GND_CTRL = HIGH
      VENT_PACE_CTRL = LOW
      Z_ATR_CTRL = LOW
      Z_VENT_CTRL = LOW
      ATR_PACE_CTRL = LOW
      ATR_GND_CTRL = HIGH
      VENT_GND_CTRL = LOW
    AAIR.Transition -> AAIR.Discharging [order 1] : after(ADAPTED_RATE - delayARP, msec)
    AAIR.Transition -> AAIR.Charging [order 2] : [ATR_CMP_DETECT == HIGH]
    AAIR.Charging -> AAIR.Transition : after(delayARP, msec)
    (default) -> AAIR.Charging
    AAIR.Discharging -> AAIR.Charging : after(delayATR_PULSEWIDTH, msec)
  state VVIR
    state Transition
      % Check for intrinsic pulse
    state Charging
      entry:
      %
      % Turn sensing on
      FRONTEND_CTRL = HIGH
      VENT_CMP_REF_PWM = VENT_SENSE
      %
      % Charging capacitor C22
      ATR_PACE_CTRL = LOW
      VENT_PACE_CTRL = LOW
      PACING_REF_PWM = VENT_AMPLITUDE
      PACE_CHARGE_CTRL = HIGH
      % Charge release of capacitor C21 into ground
      PACE_GND_CTRL = HIGH
      VENT_PACE_CTRL = LOW
      Z_ATR_CTRL = LOW
      Z_VENT_CTRL = LOW
      ATR_PACE_CTRL = LOW
      ATR_GND_CTRL = LOW
      VENT_GND_CTRL = HIGH
    state Discharging
      entry:
      %
      % Charge release of capacitor C22 into C21
      PACE_CHARGE_CTRL = LOW
      PACE_GND_CTRL = HIGH
      ATR_PACE_CTRL = LOW
      ATR_GND_CTRL = LOW
      Z_VENT_CTRL = LOW
      Z_ATR_CTRL = LOW
      VENT_GND_CTRL = LOW
      VENT_PACE_CTRL = HIGH
    VVIR.Transition -> VVIR.Discharging [order 1] : after(ADAPTED_RATE-delayVRP, msec)
    VVIR.Transition -> VVIR.Charging [order 2] : [VENT_CMP_DETECT == HIGH]
    VVIR.Charging -> VVIR.Transition : after(delayVRP, msec)
    (default) -> VVIR.Charging
    VVIR.Discharging -> VVIR.Charging : after(delayVENT_PULSEWIDTH, msec)
  ModeSelect -> AOO [order 1] : [MODE == 0]
  AOO -> ModeSelect : [MODE ~= 0]
  ModeSelect -> VOO [order 2] : [MODE == 1]
  VOO -> ModeSelect : [MODE ~= 1]
  ModeSelect -> AAI [order 3] : [MODE == 2]
  AAI -> ModeSelect : [MODE ~= 2]
  (default) -> ModeSelect : {delayINTERVAL = Lower_Rate_Interval/2,
      |  delayAV_DELAY = AV_DELAY/2,
      |  delayARP = p_ARP/2,
      |  delayVRP = p_VRP/2,
      |  delayATR_PULSEWIDTH = ATR_PULSEWIDTH/2,
      |  delayVENT_PULSEWIDTH = VENT_PULSEWIDTH/2}
  ModeSelect -> VVI [order 4] : [MODE == 3]
  VVI -> ModeSelect : [MODE ~= 3]
  ModeSelect -> AOOR [order 5] : [MODE == 4]
  AOOR -> ModeSelect : [MODE ~= 4]
  ModeSelect -> VOOR [order 6] : [MODE == 5]
  VOOR -> ModeSelect : [MODE ~= 5]
  ModeSelect -> AAIR [order 7] : [MODE == 6]
  AAIR -> ModeSelect : [MODE ~= 6]
  ModeSelect -> VVIR [order 8] : [MODE == 7]
  VVIR -> ModeSelect : [MODE ~= 7]
  data: ATR_GND_CTRL output; VENT_GND_CTRL output; VENT_PACE_CTRL output; Z_ATR_CTRL output; Z_VENT_CTRL output; PACE_GND_CTRL output; PACE_CHARGE_CTRL output; PACING_REF_PWM output; ATR_PACE_CTRL output; Lower_Rate_Interval input; HIGH local boolean =true; LOW local boolean =false; MODE input uint8; ATR_CMP_REF_PWM output; FRONTEND_CTRL output; VENT_CMP_REF_PWM output; ATR_CMP_DETECT input; VENT_CMP_DETECT input; p_ARP input single; p_VRP input single; ATR_AMPLITUDE input single; VENT_AMPLITUDE input single; ATR_PULSEWIDTH input single; VENT_PULSEWIDTH input single; VENT_SENSE input single; ATR_SENSE input single; AV_DELAY input single; ADAPTED_RATE input; delayVRP local; delayARP local; delayATR_PULSEWIDTH local; delayAV_DELAY local; delayINTERVAL local; delayVENT_PULSEWIDTH local; blue_out output; green_out output; red_out output
